simulink subsystem "TwoTanks_Sub"  (R2023b)
settings: Solver=VariableStepAuto  StartTime=0.0  StopTime=10.0  RelTol=1e-3
values from neighbouring files (symbols this model uses):
  A1 = model_params.A1    [TwoTanks_Interact_Model.m]    (also in TwoTanks_ss_model.m; init_twotanks_interact.m = Parameters.model.A1)
  A2 = model_params.A2    [TwoTanks_Interact_Model.m]    (also in TwoTanks_ss_model.m; init_twotanks_interact.m = Parameters.model.A2)
  g = model_params.g    [TwoTanks_Interact_Model.m]    (also in TwoTanks_ss_model.m; init_twotanks_interact.m = Parameters.model.g)
  gamma1 = model_params.gamma.Valve_1    [TwoTanks_Interact_Model.m]    (also in TwoTanks_ss_model.m; init_twotanks_interact.m = Parameters.model.gamma.Valve_1)
  gamma12 = model_params.gamma.Valve_12    [TwoTanks_Interact_Model.m]    (also in TwoTanks_ss_model.m; init_twotanks_interact.m = Parameters.model.gamma.Valve_12)
  gamma2 = model_params.gamma.Valve_2    [TwoTanks_Interact_Model.m]    (also in TwoTanks_ss_model.m; init_twotanks_interact.m = Parameters.model.gamma.Valve_2)
  h = Parameters.model.state_0    [init_twotanks_interact.m]
  k1 = model_params.valve_const.Valve_1    [TwoTanks_Interact_Model.m]    (also in TwoTanks_ss_model.m; init_twotanks_interact.m = Parameters.model.valve_const.Valve_1)
  k12 = model_params.valve_const.Valve_12    [TwoTanks_Interact_Model.m]    (also in TwoTanks_ss_model.m; init_twotanks_interact.m = Parameters.model.valve_const.Valve_12)
  k2 = model_params.valve_const.Valve_2    [TwoTanks_Interact_Model.m]    (also in TwoTanks_ss_model.m; init_twotanks_interact.m = Parameters.model.valve_const.Valve_2)
  kA = model_params.valve_const.Valve_A    [TwoTanks_Interact_Model.m]    (also in TwoTanks_ss_model.m; init_twotanks_interact.m = Parameters.model.valve_const.Valve_A)
  kB = model_params.valve_const.Valve_B    [TwoTanks_Interact_Model.m]    (also in TwoTanks_ss_model.m; init_twotanks_interact.m = Parameters.model.valve_const.Valve_B)
settings Model: Creator=HP  LastModifiedBy=HP

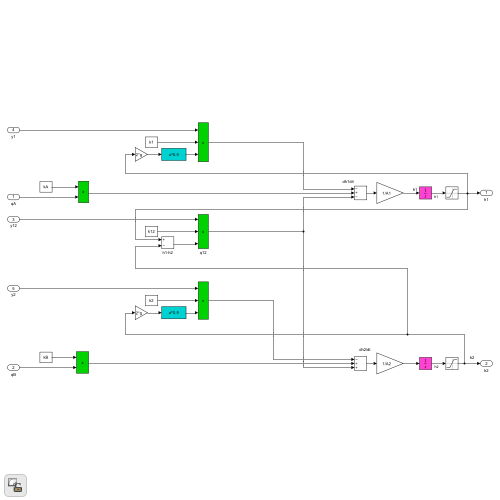
[thumbnail: Simulink's stored preview of the top-level diagram]
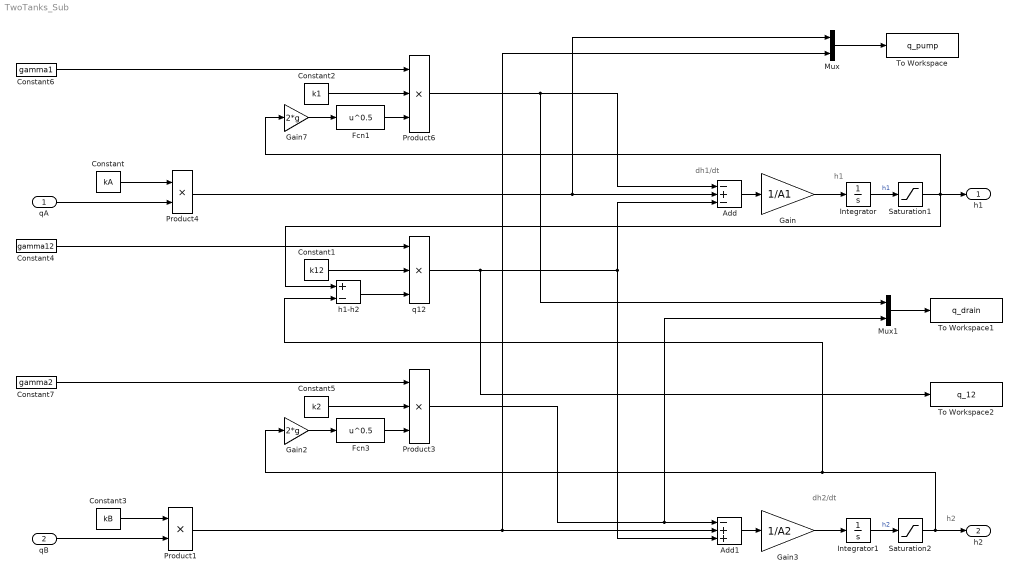
== system TwoTanks_Sub ==
  note: dh1/dt
  note: dh2/dt
  note: h2
  note: h1
  qA : Inport
  qB : Inport  Port=2
  Add : Sum  Inputs=-+-
  Add1 : Sum  Inputs=-++
  Constant : Constant  Value=kA
  Constant1 : Constant  Value=k12
  Constant2 : Constant  Value=k1
  Constant3 : Constant  Value=kB
  Constant4 : Constant  Value=gamma12
  Constant5 : Constant  Value=k2
  Constant6 : Constant  Value=gamma1
  Constant7 : Constant  Value=gamma2
  Fcn1 : Fcn  Expr=u^0.5
  Fcn3 : Fcn  Expr=u^0.5
  Gain : Gain  Gain=1/A1
  Gain2 : Gain  Gain=2*g
  Gain3 : Gain  Gain=1/A2
  Gain7 : Gain  Gain=2*g
  Integrator : Integrator  InitialCondition=h(1)
  Integrator1 : Integrator  InitialCondition=h(2)
  Mux : Mux  Inputs=2
  Mux1 : Mux  Inputs=2
  Product1 : Product  RndMeth=Zero
  Product3 : Product  Inputs=3  RndMeth=Zero
  Product4 : Product  RndMeth=Zero
  Product6 : Product  Inputs=3  RndMeth=Zero
  Saturation1 : Saturate  UpperLimit=inf  LowerLimit=0  ZeroCross=off
  Saturation2 : Saturate  UpperLimit=inf  LowerLimit=0  ZeroCross=off
  To Workspace : ToWorkspace  VariableName=q_pump  SaveFormat=Timeseries  SampleTime=-1
  To Workspace1 : ToWorkspace  VariableName=q_drain  SaveFormat=Timeseries  SampleTime=-1
  To Workspace2 : ToWorkspace  VariableName=q_12  SaveFormat=Timeseries  SampleTime=-1
  h1-h2 : Sum  Inputs=+-
  q12 : Product  Inputs=3  RndMeth=Zero
  h1 : Outport
  h2 : Outport  Port=2
  wires:
  Constant4/1 -> q12/1
  Gain3/1 -> Integrator1/1
  Product6/1 -> Add/1, Mux1/1
  Constant1/1 -> q12/2
  Constant/1 -> Product4/1
  h1-h2/1 -> q12/3
  Fcn3/1 -> Product3/3
  Saturation2/1 -> h2/1, Gain2/1, h1-h2/2
  Gain2/1 -> Fcn3/1
  Constant2/1 -> Product6/2
  Integrator/1 -> Saturation1/1  "h1"
  Product4/1 -> Add/2, Mux/1
  Add/1 -> Gain/1
  Product1/1 -> Add1/2, Mux/2
  Product3/1 -> Add1/1, Mux1/2
  Constant7/1 -> Product3/1
  Add1/1 -> Gain3/1
  Constant6/1 -> Product6/1
  Integrator1/1 -> Saturation2/1  "h2"
  Gain/1 -> Integrator/1
  q12/1 -> Add1/3, Add/3, To Workspace2/1
  Saturation1/1 -> Gain7/1, h1/1, h1-h2/1
  qA/1 -> Product4/2
  qB/1 -> Product1/2
  Fcn1/1 -> Product6/3
  Constant3/1 -> Product1/1
  Constant5/1 -> Product3/2
  Gain7/1 -> Fcn1/1
  Mux/1 -> To Workspace/1
  Mux1/1 -> To Workspace1/1
